simulink model "vision_dummy_track_sl"  (R2019a)
settings: Solver=VariableStepAuto  StartTime=0.0  StopTime=inf  RelTol=1e-3
model workspace (MAT data in the model file):
  SL_ROS_VariableLengthArrays_MaxSizes.CommonInfo.ArrayTruncateAction = 'EmitWarning'
  SL_ROS_VariableLengthArrays_MaxSizes.MsgTypeMap = containers.Map
  SL_ROS_VariableLengthArrays_MaxSizes.MsgTypeMap.serialization.keys = {'autoware_msgs/image_obj_tracked'}
  SL_ROS_VariableLengthArrays_MaxSizes.MsgTypeMap.serialization.values{1}(1).PropertyName = 'Lifespan'
  SL_ROS_VariableLengthArrays_MaxSizes.MsgTypeMap.serialization.values{1}(1).DataType = 'int32'
  SL_ROS_VariableLengthArrays_MaxSizes.MsgTypeMap.serialization.values{1}(1).MaxLength = 16
  SL_ROS_VariableLengthArrays_MaxSizes.MsgTypeMap.serialization.values{1}(2).PropertyName = 'ObjId'
  SL_ROS_VariableLengthArrays_MaxSizes.MsgTypeMap.serialization.values{1}(2).DataType = 'int32'
  SL_ROS_VariableLengthArrays_MaxSizes.MsgTypeMap.serialization.values{1}(2).MaxLength = 16
  SL_ROS_VariableLengthArrays_MaxSizes.MsgTypeMap.serialization.values{1}(3).PropertyName = 'RealData'
  SL_ROS_VariableLengthArrays_MaxSizes.MsgTypeMap.serialization.values{1}(3).DataType = 'int32'
  SL_ROS_VariableLengthArrays_MaxSizes.MsgTypeMap.serialization.values{1}(3).MaxLength = 16
  SL_ROS_VariableLengthArrays_MaxSizes.MsgTypeMap.serialization.values{1}(4).PropertyName = 'RectRanged'
  SL_ROS_VariableLengthArrays_MaxSizes.MsgTypeMap.serialization.values{1}(4).DataType = 'autoware_msgs/image_rect_ranged'
  SL_ROS_VariableLengthArrays_MaxSizes.MsgTypeMap.serialization.values{1}(4).MaxLength = 16
  SL_ROS_VariableLengthArrays_MaxSizes.MsgTypeMap.serialization.values{1}(5).PropertyName = 'Type'
  SL_ROS_VariableLengthArrays_MaxSizes.MsgTypeMap.serialization.values{1}(5).DataType = 'uint8'
  SL_ROS_VariableLengthArrays_MaxSizes.MsgTypeMap.serialization.values{1}(5).MaxLength = 128
  SL_ROS_VariableLengthArrays_MaxSizes.MsgTypeMap.serialization.uniformity = 0
  SL_ROS_VariableLengthArrays_MaxSizes.MsgTypeMap.serialization.keyType = 'char'
  SL_ROS_VariableLengthArrays_MaxSizes.MsgTypeMap.serialization.valueType = 'any'
undefined symbols (not defined in the file): Header, Lifespan, ObjId, RealData, RectRanged, RectRanged_SL_Info, TotalNum, Type, Type_SL_Info
libraries: robotlib x3
settings Model: Creator=handai  LastModifiedBy=root
settings DataIOCC: ReturnWorkspaceOutputs=off
settings DebuggingCC: ArithmeticOperatorsInVariantConditions=warning

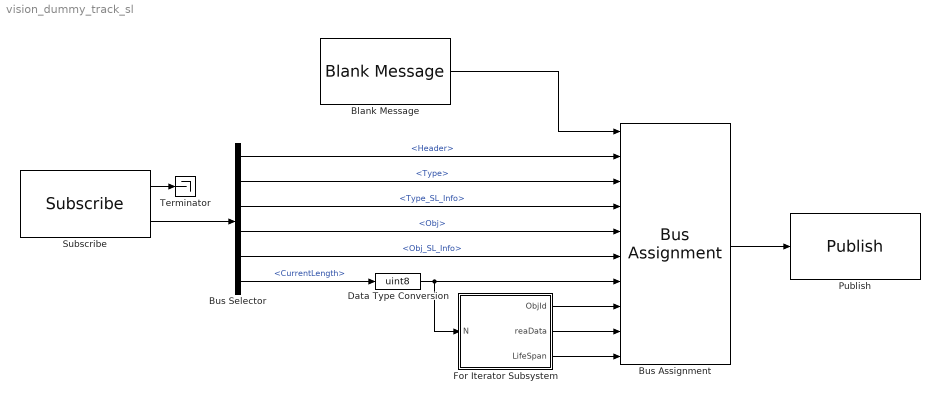
== system vision_dummy_track_sl ==
  Blank Message : robotlib/Blank Message  messageClass=Message  entityType=autoware_msgs/ImageObjTracked  messageType=autoware_msgs/ImageObjTracked  SampleTime=inf
      settings: SourceProductBaseCode=RO
  Bus Assignment : BusAssignment  AssignedSignals=Header,Type,Type_SL_Info,RectRanged,RectRanged_SL_Info,TotalNum,ObjId,RealData,Lifespan
  Bus Selector : BusSelector  OutputSignals=Header,Type,Type_SL_Info,Obj,Obj_SL_Info,Obj_SL_Info.CurrentLength
  Data Type Conversion : DataTypeConversion  OutDataTypeStr=uint8
  For Iterator Subsystem : Subsystem  TreatAsAtomicUnit=on
  Publish : robotlib/Publish  topicSource=Specify your own  topic=/obj_car/image_obj_tracked  messageType=autoware_msgs/ImageObjTracked  messageQueueLength=1
      settings: SourceProductBaseCode=RO
  Subscribe : robotlib/Subscribe  topicSource=Specify your own  topic=/obj_car/image_obj_ranged  messageType=autoware_msgs/ImageObjTracked  sampleTime=-1  messageQueueLength=1
      settings: SourceProductBaseCode=RO
  Terminator : Terminator
  wires:
  Blank Message/1 -> Bus Assignment/1
  Subscribe/2 -> Bus Selector/1
  Bus Selector/1 -> Bus Assignment/2  "<Header>"
  Bus Selector/2 -> Bus Assignment/3  "<Type>"
  Bus Selector/3 -> Bus Assignment/4  "<Type_SL_Info>"
  Bus Selector/6 -> Data Type Conversion/1  "<CurrentLength>"
  Bus Selector/4 -> Bus Assignment/5  "<Obj>"
  Data Type Conversion/1 -> Bus Assignment/7, For Iterator Subsystem/1(N)
  Subscribe/1 -> Terminator/1
  Bus Selector/5 -> Bus Assignment/6  "<Obj_SL_Info>"
  For Iterator Subsystem/1(ObjId) -> Bus Assignment/8
  For Iterator Subsystem/2(reaData) -> Bus Assignment/9
  For Iterator Subsystem/3(LifeSpan) -> Bus Assignment/10
  Bus Assignment/1 -> Publish/1

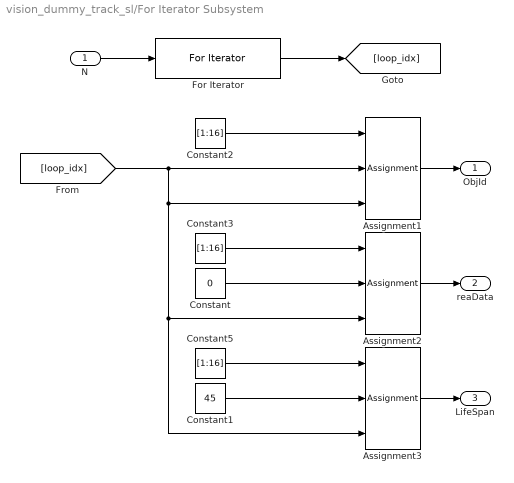
== system vision_dummy_track_sl/For Iterator Subsystem ==
  N : Inport
  Assignment1 : Assignment  DiagnosticForDimensions=Warning  IndexOptions=Index vector (port)  Indices=1  OutputSizes=1
  Assignment2 : Assignment  DiagnosticForDimensions=Warning  IndexOptions=Index vector (port)  Indices=1  OutputSizes=1
  Assignment3 : Assignment  DiagnosticForDimensions=Warning  IndexOptions=Index vector (port)  Indices=1  OutputSizes=1
  Constant : Constant  Value=0  OutDataTypeStr=int32
  Constant1 : Constant  Value=45  OutDataTypeStr=int32
  Constant2 : Constant  Value=[1:16]  OutDataTypeStr=int32
  Constant3 : Constant  Value=[1:16]  OutDataTypeStr=int32
  Constant5 : Constant  Value=[1:16]  OutDataTypeStr=int32
  For Iterator : ForIterator  ResetStates=reset  IterationSource=external
  ObjId : Outport
  reaData : Outport  Port=2
  LifeSpan : Outport  Port=3
  wires:
  Assignment1/1 -> ObjId/1
  For Iterator/1 -> [loop_idx]
  N/1 -> For Iterator/1
  Constant2/1 -> Assignment1/1
  Constant3/1 -> Assignment2/1
  Assignment2/1 -> reaData/1
  Constant/1 -> Assignment2/2
  Constant5/1 -> Assignment3/1
  Constant1/1 -> Assignment3/2
  [loop_idx] -> Assignment3/3, Assignment2/3, Assignment1/3, Assignment1/2
  Assignment3/1 -> LifeSpan/1
